simulink model "LMS_cs"  (R2023a)
settings: Solver=ode5  StartTime=0.0  StopTime=inf  FixedStep=1/200  RelTol=1e-3
PreLoadFcn:
  | mbxruntime.callbacks.PreLoadFcn(bdroot);
PostLoadFcn:
  | mbxruntime.callbacks.PostLoadFcn(bdroot);
InitFcn:
  | mbxruntime.callbacks.InitFcn(bdroot);
StartFcn:
  | mbxruntime.callbacks.StartFcn(bdroot);
StopFcn:
  | mbxruntime.callbacks.StopFcn(bdroot);
model workspace (MAT data in the model file):
  mbox_table : object (value not decoded)
  model_closed = 0
  sim_status = 0
undefined symbols (not defined in the file or in its folder): DiscIntNeverNeededParam, WheelL0, WheelL1, WheelR0, WheelR1
libraries: simulink x462, simulink_extras x117, PreScanSimulinkLibrary x33, PreScanUsefulBlocks x6, instrumentseriallib x5, simulink_need_slupdate x1
(part 62 of 68)

== system LMS_cs/BMW_X5_SUV_7/Dynamics_Simple_3D/Chassis/Bicycle_model_[XYZ]/X_Motion/BrakeSystem ==
  vx_[ms-1] : Inport
  BrakePressure_[bar] : Inport  Port=2
  Gain : Gain  Gain=1/p.Rw
  Saturation : Saturate  UpperLimit=p.PBrakeMax  LowerLimit=0
  Saturation1 : Saturate  UpperLimit=5/15  LowerLimit=-5/15
  Sign : Signum
  "[ms-1] 2 [rads-1]" : Gain  Gain=1/p.Rw  SaturateOnIntegerOverflow=on  OutDataTypeStr=Inherit: Same as input  ParamDataTypeStr=Inherit: Same as input
  braking Q factor : Gain  Gain=p.Qfac  SaturateOnIntegerOverflow=on  OutDataTypeStr=Inherit: Same as input  ParamDataTypeStr=Inherit: Same as input
  signed load1 : Product  InputSameDT=on  SaturateOnIntegerOverflow=on  OutDataTypeStr=Inherit: Same as first input
  BrakeForce : Outport
  BrakeTorqueAbs : Outport  Port=2
  wires:
  Gain/1 -> signed load1/1
  signed load1/1 -> BrakeForce/1
  Sign/1 -> signed load1/2  "sign"
  "[ms-1] 2 [rads-1]"/1 -> Saturation1/1
  Saturation1/1 -> Sign/1
  vx_[ms-1]/1 -> "[ms-1] 2 [rads-1]"/1
  Saturation/1 -> braking Q factor/1
  BrakePressure_[bar]/1 -> Saturation/1
  braking Q factor/1 -> Gain/1, BrakeTorqueAbs/1

== system LMS_cs/BMW_X5_SUV_7/Dynamics_Simple_3D/Chassis/Bicycle_model_[XYZ]/X_Motion/Configurable Subsystem ==
  In1 : Inport
  In2 : Inport  Port=2
  In3 : Inport  Port=3
  Integrator : Integrator  ExternalReset=level  InitialConditionSource=external
  Out1 : Outport
  wires:
  In1/1 -> Integrator/1
  In2/1 -> Integrator/2
  In3/1 -> Integrator/3
  Integrator/1 -> Out1/1

== system LMS_cs/BMW_X5_SUV_7/Dynamics_Simple_3D/Chassis/Bicycle_model_[XYZ]/X_Motion/Configurable Subsystem1 ==
  In1 : Inport
  Torsional damping : TransferFcn  Denominator=[0.1 1]
  Out1 : Outport
  wires:
  In1/1 -> Torsional damping/1
  Torsional damping/1 -> Out1/1

== system LMS_cs/BMW_X5_SUV_7/Dynamics_Simple_3D/Chassis/Bicycle_model_[XYZ]/X_Motion/Max RPM and zero- velocity detection ==
  note: Zero velocity detection
  note: Set to zero after infinite small time-step
  ax : Inport
  Drive Torque : Inport  Port=2
  Slope Torque : Inport  Port=3
  Brake Torque : Inport  Port=4
  v0 : Inport  Port=5
  vx : Inport  Port=6
  Abs : Abs  SaturateOnIntegerOverflow=off
  Abs1 : Abs  SaturateOnIntegerOverflow=off
  Compare To Zero : simulink/Logic and Bit Operations/Compare To Zero  relop=<=  OutDataTypeStr=boolean  ZeroCross=off
  Compare To Zero1 : simulink/Logic and Bit Operations/Compare To Zero  relop=>=  OutDataTypeStr=boolean  ZeroCross=off
  Compare To Zero2 : simulink/Logic and Bit Operations/Compare To Zero  relop=>=  OutDataTypeStr=boolean  ZeroCross=off
  Compare To Zero3 : simulink/Logic and Bit Operations/Compare To Zero  relop=<=  OutDataTypeStr=boolean  ZeroCross=off
  Configurable Subsystem : Subsystem  BlockChoice=Step  mask{ComputationMode=ComputationMode}
      mask prompts: ComputationMode "Compuation mode:"
      mask init:
      | SetComputationMode(gcb,ComputationMode);
      settings: AttributesFormatString=%<BlockChoice>  OpenFcn=BringToFront(gcb);  MemberBlocks=Discrete Step,Step
      settings: TemplateBlock=|
      | PreScanSimulinkLibrary/Configurable Subsystems/Step Function/Configurable
      | Subsystem
  Constant : Constant
  Constant1 : Constant
  Logical Operator : Logic  AllPortsSameDT=off  OutDataTypeStr=boolean
  Logical Operator1 : Logic  AllPortsSameDT=off  OutDataTypeStr=boolean
  Logical Operator2 : Logic  Operator=NOT  AllPortsSameDT=off  OutDataTypeStr=boolean
  Logical Operator3 : Logic  AllPortsSameDT=off  OutDataTypeStr=boolean
  Logical Operator4 : Logic  Operator=OR  AllPortsSameDT=off  OutDataTypeStr=boolean
  Memory : Memory
  Memory1 : Memory
  Memory2 : Memory
  Product : Product  RndMeth=Zero
  Relational Operator : RelationalOperator  Operator=<  OutDataTypeStr=boolean  InputSameDT=off
  SR-Memory : Subsystem
  Sum : Sum  Inputs=|-+
  Sum3 : Sum  InputSameDT=on  SaturateOnIntegerOverflow=on  OutDataTypeStr=Inherit: Same as first input
  Switch : Switch  Criteria=u2 ~= 0  Threshold=0.5  SaturateOnIntegerOverflow=off  InputSameDT=off
  ax is 0 : Constant  Value=0
  ax_out : Outport
  vx_reset : Outport  Port=2
  x0 : Outport  Port=3
  wires:
  Abs/1 -> Relational Operator/1
  Sum3/1 -> Abs/1
  Drive Torque/1 -> Sum3/1
  Slope Torque/1 -> Sum3/2
  Memory1/1 -> vx_reset/1  "vx"
  ax/1 -> Switch/1  "ax"
  Configurable Subsystem/1(Out1) -> Product/2
  Product/1 -> x0/1
  v0/1 -> Product/1
  Constant1/1 -> Sum/2
  ax is 0/1 -> Switch/3
  Sum/1 -> Switch/2
  Switch/1 -> ax_out/1
  SR-Memory/1(Out) -> Memory1/1, Sum/1
  Logical Operator2/1 -> SR-Memory/3(Reset)
  Constant/1 -> SR-Memory/1(Signal)
  Logical Operator1/1 -> SR-Memory/2(Set)
  Relational Operator/1 -> Logical Operator2/1, Logical Operator1/2
  Brake Torque/1 -> Abs1/1
  Abs1/1 -> Relational Operator/2
  Logical Operator/1 -> Logical Operator4/1  "zero-crossing forward"
  Compare To Zero1/1 -> Logical Operator/2
  Compare To Zero/1 -> Logical Operator/1
  Memory/1 -> Compare To Zero1/1
  Logical Operator3/1 -> Logical Operator4/2  "zero-crossing backward"
  Compare To Zero3/1 -> Logical Operator3/2
  Compare To Zero2/1 -> Logical Operator3/1
  Memory2/1 -> Compare To Zero3/1
  vx/1 -> Memory/1, Memory2/1, Compare To Zero2/1, Compare To Zero/1  "vx"
  Logical Operator4/1 -> Logical Operator1/1

== system LMS_cs/BMW_X5_SUV_7/Dynamics_Simple_3D/Chassis/Bicycle_model_[XYZ]/X_Motion/No contact rear wheels ==
  ForceIn [N] : Inport
  Compare To Zero : simulink/Logic and Bit Operations/Compare To Zero  relop=~=  OutDataTypeStr=boolean  ZeroCross=off
  Compare To Zero1 : simulink/Logic and Bit Operations/Compare To Zero  relop=~=  OutDataTypeStr=boolean  ZeroCross=off
  Constant : Constant  Value=0
  Logical Operator : Logic  AllPortsSameDT=off  OutDataTypeStr=boolean
  Switch : Switch  Criteria=u2 ~= 0  SaturateOnIntegerOverflow=off  InputSameDT=off
  ForceOut [N] : Outport
  wires:
  Switch/1 -> ForceOut [N]/1
  ForceIn [N]/1 -> Switch/1
  Logical Operator/1 -> Switch/2
  Compare To Zero1/1 -> Logical Operator/2
  Compare To Zero/1 -> Logical Operator/1
  [penetrationrearright] -> Compare To Zero1/1
  [penetrationrearleft] -> Compare To Zero/1
  Constant/1 -> Switch/3

== system LMS_cs/BMW_X5_SUV_7/Dynamics_Simple_3D/Chassis/Bicycle_model_[XYZ]/X_Motion/No contact wheels ==
  ForceIn [N] : Inport
  Brake repartition : Fcn  Expr=u(1) * (u(2)/4)
  Compare To Zero{,1..3} (4 alike) : simulink/Logic and Bit Operations/Compare To Zero  relop=~=  OutDataTypeStr=boolean  ZeroCross=off
  Mux : Mux  Inputs=[1 1 ]
  Sum : Sum  Inputs=++++  OutDataTypeStr=double
  ForceOut [N] : Outport
  wires:
  Brake repartition/1 -> ForceOut [N]/1
  Mux/1 -> Brake repartition/1
  Compare To Zero1/1 -> Sum/4
  Compare To Zero/1 -> Sum/3
  Compare To Zero3/1 -> Sum/2
  Compare To Zero2/1 -> Sum/1
  [penetrationfrontright] -> Compare To Zero3/1
  [penetrationfrontleft] -> Compare To Zero2/1
  ForceIn [N]/1 -> Mux/1
  Sum/1 -> Mux/2
  [penetrationrearright] -> Compare To Zero1/1
  [penetrationrearleft] -> Compare To Zero/1

== system LMS_cs/BMW_X5_SUV_7/Dynamics_Simple_3D/Chassis/Bicycle_model_[XYZ]/X_Motion/Slope Force ==
  slope_[rad] : Inport
  Fcn5 : Fcn  Expr=p.m*p.g*sin(u(1))
  SlopeForce_[N] : Outport
  wires:
  Fcn5/1 -> SlopeForce_[N]/1  "SlopeForce_[N]"
  slope_[rad]/1 -> Fcn5/1  "slope_[rad]"

== system LMS_cs/BMW_X5_SUV_7/Dynamics_Simple_3D/Chassis/Bicycle_model_[XYZ]/Y & Yaw_Motion/Configurable Subsystem ==
  In1 : Inport
  In2 : Inport  Port=2
  Integrator : Integrator  ExternalReset=level
  Out1 : Outport
  wires:
  In1/1 -> Integrator/1
  In2/1 -> Integrator/2
  Integrator/1 -> Out1/1

== system LMS_cs/BMW_X5_SUV_7/Dynamics_Simple_3D/Chassis/Bicycle_model_[XYZ]/Y & Yaw_Motion/Configurable Subsystem1 ==
  In1 : Inport
  In2 : Inport  Port=2
  Integrator : Integrator  ExternalReset=level
  Out1 : Outport
  wires:
  In1/1 -> Integrator/1
  In2/1 -> Integrator/2
  Integrator/1 -> Out1/1

== system LMS_cs/BMW_X5_SUV_7/Dynamics_Simple_3D/Chassis/Bicycle_model_[XYZ]/Y & Yaw_Motion/Configurable Subsystem2 ==
  In1 : Inport
  Integrator : Integrator
  Out1 : Outport
  wires:
  In1/1 -> Integrator/1
  Integrator/1 -> Out1/1

== system LMS_cs/BMW_X5_SUV_7/Dynamics_Simple_3D/Chassis/Bicycle_model_[XYZ]/Z, Pitch_Motion & Roll_Motion/Configurable Subsystem ==
  In1 : Inport
  Integrator : Integrator  LimitOutput=on  UpperSaturationLimit=25*pi/180  LowerSaturationLimit=-25*pi/180
  Out1 : Outport
  wires:
  In1/1 -> Integrator/1
  Integrator/1 -> Out1/1

== system LMS_cs/BMW_X5_SUV_7/Dynamics_Simple_3D/Chassis/Bicycle_model_[XYZ]/Z, Pitch_Motion & Roll_Motion/Configurable Subsystem1 ==
  In1 : Inport
  Integrator : Integrator
  Out1 : Outport
  wires:
  In1/1 -> Integrator/1
  Integrator/1 -> Out1/1

== system LMS_cs/BMW_X5_SUV_7/Dynamics_Simple_3D/Chassis/Bicycle_model_[XYZ]/Z, Pitch_Motion & Roll_Motion/Configurable Subsystem2 ==
  In1 : Inport
  Integrator : Integrator
  Out1 : Outport
  wires:
  In1/1 -> Integrator/1
  Integrator/1 -> Out1/1

== system LMS_cs/BMW_X5_SUV_7/Dynamics_Simple_3D/Chassis/Bicycle_model_[XYZ]/Z, Pitch_Motion & Roll_Motion/Configurable Subsystem3 ==
  In1 : Inport
  Integrator : Integrator
  Out1 : Outport
  wires:
  In1/1 -> Integrator/1
  Integrator/1 -> Out1/1

== system LMS_cs/BMW_X5_SUV_7/Dynamics_Simple_3D/Chassis/Bicycle_model_[XYZ]/Z, Pitch_Motion & Roll_Motion/Configurable Subsystem4 ==
  In1 : Inport
  Integrator : Integrator
  Out1 : Outport
  wires:
  In1/1 -> Integrator/1
  Integrator/1 -> Out1/1

== system LMS_cs/BMW_X5_SUV_7/Dynamics_Simple_3D/Chassis/Bicycle_model_[XYZ]/Z, Pitch_Motion & Roll_Motion/Configurable Subsystem5 ==
  In1 : Inport
  Derivative : Derivative
  Out1 : Outport
  wires:
  In1/1 -> Derivative/1
  Derivative/1 -> Out1/1

== system LMS_cs/BMW_X5_SUV_7/Dynamics_Simple_3D/Chassis/Bicycle_model_[XYZ]/Z, Pitch_Motion & Roll_Motion/Configurable Subsystem6 ==
  In1 : Inport
  Derivative : Derivative
  Out1 : Outport
  wires:
  In1/1 -> Derivative/1
  Derivative/1 -> Out1/1

== system LMS_cs/BMW_X5_SUV_7/Dynamics_Simple_3D/Chassis/Bicycle_model_[XYZ]/Z, Pitch_Motion & Roll_Motion/Configurable Subsystem7 ==
  In1 : Inport
  Derivative : Derivative
  Out1 : Outport
  wires:
  In1/1 -> Derivative/1
  Derivative/1 -> Out1/1

== system LMS_cs/BMW_X5_SUV_7/Dynamics_Simple_3D/Chassis/Bicycle_model_[XYZ]/Z, Pitch_Motion & Roll_Motion/Configurable Subsystem8 ==
  In1 : Inport
  Derivative : Derivative
  Out1 : Outport
  wires:
  In1/1 -> Derivative/1
  Derivative/1 -> Out1/1

== system LMS_cs/BMW_X5_SUV_7/Dynamics_Simple_3D/Chassis/Bicycle_model_[XYZ]/Z, Pitch_Motion & Roll_Motion/Configurable Subsystem9 ==
  In1 : Inport
  Derivative : Derivative
  Out1 : Outport
  wires:
  In1/1 -> Derivative/1
  Derivative/1 -> Out1/1

== system LMS_cs/BMW_X5_SUV_7/Dynamics_Simple_3D/Chassis/Bicycle_model_[XYZ]/Z_Motion unsprung mass/Configurable Subsystem ==
  In1 : Inport
  Derivative : Derivative
  Out1 : Outport
  wires:
  In1/1 -> Derivative/1
  Derivative/1 -> Out1/1

== system LMS_cs/BMW_X5_SUV_7/Dynamics_Simple_3D/Chassis/Bicycle_model_[XYZ]/Z_Motion unsprung mass/Configurable Subsystem1 ==
  In1 : Inport
  Integrator : Integrator
  Out1 : Outport
  wires:
  In1/1 -> Integrator/1
  Integrator/1 -> Out1/1

== system LMS_cs/BMW_X5_SUV_7/Dynamics_Simple_3D/Chassis/Bicycle_model_[XYZ]/Z_Motion unsprung mass/Configurable Subsystem10 ==
  In1 : Inport
  Derivative : Derivative
  Out1 : Outport
  wires:
  In1/1 -> Derivative/1
  Derivative/1 -> Out1/1

== system LMS_cs/BMW_X5_SUV_7/Dynamics_Simple_3D/Chassis/Bicycle_model_[XYZ]/Z_Motion unsprung mass/Configurable Subsystem11 ==
  In1 : Inport
  Derivative : Derivative
  Out1 : Outport
  wires:
  In1/1 -> Derivative/1
  Derivative/1 -> Out1/1

== system LMS_cs/BMW_X5_SUV_7/Dynamics_Simple_3D/Chassis/Bicycle_model_[XYZ]/Z_Motion unsprung mass/Configurable Subsystem2 ==
  In1 : Inport
  Integrator : Integrator
  Out1 : Outport
  wires:
  In1/1 -> Integrator/1
  Integrator/1 -> Out1/1

== system LMS_cs/BMW_X5_SUV_7/Dynamics_Simple_3D/Chassis/Bicycle_model_[XYZ]/Z_Motion unsprung mass/Configurable Subsystem3 ==
  In1 : Inport
  Integrator : Integrator
  Out1 : Outport
  wires:
  In1/1 -> Integrator/1
  Integrator/1 -> Out1/1

== system LMS_cs/BMW_X5_SUV_7/Dynamics_Simple_3D/Chassis/Bicycle_model_[XYZ]/Z_Motion unsprung mass/Configurable Subsystem4 ==
  In1 : Inport
  Integrator : Integrator
  Out1 : Outport
  wires:
  In1/1 -> Integrator/1
  Integrator/1 -> Out1/1

== system LMS_cs/BMW_X5_SUV_7/Dynamics_Simple_3D/Chassis/Bicycle_model_[XYZ]/Z_Motion unsprung mass/Configurable Subsystem5 ==
  In1 : Inport
  Integrator : Integrator
  Out1 : Outport
  wires:
  In1/1 -> Integrator/1
  Integrator/1 -> Out1/1

== system LMS_cs/BMW_X5_SUV_7/Dynamics_Simple_3D/Chassis/Bicycle_model_[XYZ]/Z_Motion unsprung mass/Configurable Subsystem6 ==
  In1 : Inport
  Integrator : Integrator
  Out1 : Outport
  wires:
  In1/1 -> Integrator/1
  Integrator/1 -> Out1/1

== system LMS_cs/BMW_X5_SUV_7/Dynamics_Simple_3D/Chassis/Bicycle_model_[XYZ]/Z_Motion unsprung mass/Configurable Subsystem7 ==
  In1 : Inport
  Integrator : Integrator
  Out1 : Outport
  wires:
  In1/1 -> Integrator/1
  Integrator/1 -> Out1/1

== system LMS_cs/BMW_X5_SUV_7/Dynamics_Simple_3D/Chassis/Bicycle_model_[XYZ]/Z_Motion unsprung mass/Configurable Subsystem8 ==
  In1 : Inport
  Integrator : Integrator
  Out1 : Outport
  wires:
  In1/1 -> Integrator/1
  Integrator/1 -> Out1/1

== system LMS_cs/BMW_X5_SUV_7/Dynamics_Simple_3D/Chassis/Bicycle_model_[XYZ]/Z_Motion unsprung mass/Configurable Subsystem9 ==
  In1 : Inport
  Derivative : Derivative
  Out1 : Outport
  wires:
  In1/1 -> Derivative/1
  Derivative/1 -> Out1/1

== system LMS_cs/BMW_X5_SUV_7/Dynamics_Simple_3D/Chassis/FrontTyre/AlphaFront/Enabled Subsystem ==
  In : Inport
  Enable : EnablePort  PropagateVarSize=During execution
  AlphaFront : Fcn  Expr=-atan( (u(2)+u(3)*p.a)/u(1) )
  Alpha : Outport  OutputWhenDisabled=reset  InitialOutput=[0]
  wires:
  AlphaFront/1 -> Alpha/1
  In/1 -> AlphaFront/1

== system LMS_cs/BMW_X5_SUV_7/Dynamics_Simple_3D/Chassis/RearTyre/AlphaRear/Enabled Subsystem ==
  In : Inport
  Enable : EnablePort  PropagateVarSize=During execution
  AlphaRear : Fcn  Expr=-atan( (u(2)-u(3)*p.b)/u(1) )
  Alpha : Outport  OutputWhenDisabled=reset  InitialOutput=[0]
  wires:
  AlphaRear/1 -> Alpha/1
  In/1 -> AlphaRear/1

== system LMS_cs/BMW_X5_SUV_7/PreScan_Contact_Sensor/Vehicle Local to World/state2FullState/limit roll/Substitute 90 & 270 deg (and its plurals) ==
  Angle [rad] : Inport
  270 deg detection : simulink/Model Verification/Check  Static Gap  Description=u <= 269.5 || 270.5 <= u  max=270.5  max_included=on  min=269.5  min_included=on  enabled=on  stopWhenAssertionFail=off  export=on  icon=graphic
  90 deg detection : simulink/Model Verification/Check  Static Gap  Description=u <= 89.5 || 90.5 <= u  max=90.5  max_included=on  min=89.5  min_included=on  enabled=on  stopWhenAssertionFail=off  export=on  icon=graphic
  Angle 0-360 deg limiter : Subsystem
  Degrees to Radians : simulink_extras/Transformations/Degrees to Radians
  Radians to Degrees : simulink_extras/Transformations/Radians to Degrees
  Substitution Value : Constant  Value=269.5
  Substitution Value : Constant  Value=89.5
  Switch : Switch  Threshold=0.5  SaturateOnIntegerOverflow=off  InputSameDT=off
  Switch1 : Switch  Threshold=0.5  SaturateOnIntegerOverflow=off  InputSameDT=off
  Subst Angle [rad] : Outport
  wires:
  Angle [rad]/1 -> Radians to Degrees/1
  Degrees to Radians/1 -> Subst Angle [rad]/1
  Radians to Degrees/1 -> Angle 0-360 deg limiter/1(Angle [deg])
  Switch1/1 -> Degrees to Radians/1
  Substitution Value/1 -> Switch1/3
  270 deg detection/1 -> Switch1/2
  Switch/1 -> Switch1/1, 270 deg detection/1
  Substitution Value/1 -> Switch/3
  90 deg detection/1 -> Switch/2
  Angle 0-360 deg limiter/1(LimAngle [deg]) -> 90 deg detection/1, Switch/1

== system LMS_cs/BMW_X5_SUV_8/Dynamics_Simple_3D/Chassis/Bicycle_model_[XYZ]/RoadContact/Penetration depth ==
  TyreInfo_in : Inport
  Bus Selector1 : BusSelector  OutputSignals=TireFL.cp0.penetrationdepth,TireFL.cp0.normal.z,TireFL.cp1.penetrationdepth,TireFL.cp1.normal.z,TireFL.cp2.penetrationdepth,TireFL.cp2.normal.z,TireFL.cp3.penetrationdepth,TireFL.cp3.normal.z,TireFR.cp0.penetrationdepth,TireFR.cp0.normal.z,TireFR.cp1.penetrationdepth,TireFR.cp1.normal.z,TireFR.cp2.penetrationdepth,TireFR.cp2.normal.z,TireFR.cp3.penetrationdepth,TireFR.cp3.normal.z,TireRL.cp0.penetrationdepth,TireRL.cp0.normal.z,TireRL.cp1.penetrationdepth,TireRL.cp1.normal.z,TireRL.cp2.penetrationdepth,TireRL.cp2.normal.z,TireRL.cp3.penetrationdepth,TireRL.cp3.normal.z,TireRR.cp0.penetrationdepth,TireRR.cp0.normal.z,TireRR.cp1.penetrationdepth,TireRR.cp1.normal.z,TireRR.cp2.penetrationdepth,TireRR.cp2.normal.z,TireRR.cp3.penetrationdepth,TireRR.cp3.normal.z
  Fcn{,1..15} (16 alike) : Fcn  Expr=u(1)*u(2)
  MinMax{1..4} (4 alike) : MinMax
  Mux{1..4} (4 alike) : Mux
  Mux{5..20} (16 alike) : Mux  Inputs=2
  Saturation{1..4} (4 alike) : Saturate  UpperLimit=0  LowerLimit=-inf
  depth_FL [m] : Outport
  depth_FR [m] : Outport  Port=2
  depth_RL [m] : Outport  Port=3
  depth_RR [m] : Outport  Port=4
  wires:
  Fcn15/1 -> Mux4/4
  Fcn14/1 -> Mux4/3
  Fcn13/1 -> Mux4/2
  Fcn12/1 -> Mux4/1
  Fcn11/1 -> Mux2/4
  Fcn10/1 -> Mux2/3
  Fcn9/1 -> Mux2/2
  Fcn8/1 -> Mux2/1
  Mux15/1 -> Fcn15/1
  Mux14/1 -> Fcn14/1
  Mux13/1 -> Fcn13/1
  Mux20/1 -> Fcn12/1
  Mux19/1 -> Fcn11/1
  Mux18/1 -> Fcn10/1
  Mux17/1 -> Fcn9/1
  Mux16/1 -> Fcn8/1
  Fcn7/1 -> Mux1/4
  Fcn6/1 -> Mux1/3
  Fcn5/1 -> Mux1/2
  Fcn4/1 -> Mux1/1
  Fcn3/1 -> Mux3/4
  Fcn2/1 -> Mux3/3
  Fcn1/1 -> Mux3/2
  Fcn/1 -> Mux3/1
  Mux12/1 -> Fcn7/1
  Mux11/1 -> Fcn6/1
  Mux10/1 -> Fcn5/1
  Mux9/1 -> Fcn4/1
  Mux8/1 -> Fcn3/1
  Mux7/1 -> Fcn2/1
  Mux6/1 -> Fcn1/1
  Mux5/1 -> Fcn/1
  MinMax1/1 -> Saturation2/1
  Mux1/1 -> MinMax1/1
  MinMax2/1 -> Saturation3/1
  Mux2/1 -> MinMax2/1
  MinMax4/1 -> Saturation1/1
  Bus Selector1/32 -> Mux15/2  "<z>"
  Bus Selector1/31 -> Mux15/1  "<penetrationdepth>"
  Bus Selector1/30 -> Mux14/2  "<z>"
  Bus Selector1/29 -> Mux14/1  "<penetrationdepth>"
  Bus Selector1/28 -> Mux13/2  "<z>"
  Bus Selector1/27 -> Mux13/1  "<penetrationdepth>"
  Bus Selector1/26 -> Mux20/2  "<z>"
  Bus Selector1/25 -> Mux20/1  "<penetrationdepth>"
  Bus Selector1/24 -> Mux19/2  "<z>"
  Bus Selector1/23 -> Mux19/1  "<penetrationdepth>"
  Bus Selector1/22 -> Mux18/2  "<z>"
  Bus Selector1/21 -> Mux18/1  "<penetrationdepth>"
  Bus Selector1/20 -> Mux17/2  "<z>"
  Bus Selector1/19 -> Mux17/1  "<penetrationdepth>"
  Bus Selector1/18 -> Mux16/2  "<z>"
  Bus Selector1/17 -> Mux16/1  "<penetrationdepth>"
  Bus Selector1/16 -> Mux12/2  "<z>"
  Bus Selector1/15 -> Mux12/1  "<penetrationdepth>"
  Bus Selector1/14 -> Mux11/2  "<z>"
  Bus Selector1/13 -> Mux11/1  "<penetrationdepth>"
  Bus Selector1/12 -> Mux10/2  "<z>"
  Bus Selector1/11 -> Mux10/1  "<penetrationdepth>"
  Bus Selector1/10 -> Mux9/2  "<z>"
  Bus Selector1/9 -> Mux9/1  "<penetrationdepth>"
  Bus Selector1/8 -> Mux8/2  "<z>"
  Bus Selector1/7 -> Mux8/1  "<penetrationdepth>"
  Bus Selector1/6 -> Mux7/2  "<z>"
  Bus Selector1/5 -> Mux7/1  "<penetrationdepth>"
  Bus Selector1/4 -> Mux6/2  "<z>"
  Bus Selector1/3 -> Mux6/1  "<penetrationdepth>"
  Bus Selector1/2 -> Mux5/2  "<z>"
  Bus Selector1/1 -> Mux5/1  "<penetrationdepth>"
  Mux4/1 -> MinMax3/1
  MinMax3/1 -> Saturation4/1
  Mux3/1 -> MinMax4/1
  Saturation1/1 -> depth_FL [m]/1
  Saturation2/1 -> depth_FR [m]/1
  TyreInfo_in/1 -> Bus Selector1/1
  Saturation3/1 -> depth_RL [m]/1
  Saturation4/1 -> depth_RR [m]/1

== system LMS_cs/BMW_X5_SUV_8/Dynamics_Simple_3D/Chassis/Bicycle_model_[XYZ]/RoadContact/RoadGeometry ==
  TyreInfo_in : Inport
  Calc_banking : Subsystem
  Calc_slope : Subsystem
  Calc_z : Subsystem
  DocBlock : simulink/Model-Wide Utilities/DocBlock  DocumentType=Text
      content=|
      | This block determines, based on the z-coordinates of the road in
      | correspondence of the contact points,
      | - the z-coordinate of the road in correspondence of the middle point of the
      |   vehicle (z);
      | - the slope angle of the road (alpha, positive when downhill);
      | - the banking angle of the road (beta, positive when counter-clockwise when
      |   looking from the front of the vehicle).
      |
      | For every wheel there are 4 contact points (cp0, cp1, cp2, cp3) defined in
      | TyreInfo_in. Not all 4 contact points reports always a value, depending on
      | different conditions there might be contact points that do not report a
      | value. These points report in this case to 0. If the tyre is lifted from
      | the road, all contact points report 0. Because of this reason, the
      | value of the contact point that reports the largest negative value of the
      | penetration depth is used. If all values of the penetration depth are 0,
      | then a maximum gradient is applied to avoid jumps to 0 in the z signal.
      | The maximum gradient is fixed to -6 [m/s^2], this value is large enough for
      | a vehicle driving at 30 [m/s] downhill on a gradient of 20 [%]. Further, a
      | first order low pass linear filter with a bandwidth of 1 [Hz] is applied.
      | This filter removes high frequencies components in the signal, when one
      | wheel is lifted (e.g. drive in a corner with a large lateral acceleration).
      | The bandwidth of 1 [Hz] is large enough to include the main frequencies
      | that occurr in the vehicle roll, pitch and vertical movements.
      |
      | z, slope and banking are determined as follows:
      |
      | z        = (+ zFL + zFR + zRL + zRR) / 4            (Calc_z)
      | slope    = (- zFL - zFR + zRL + zRR) / (2*p.l)      (Calc_slope)
      | banking  = (+ zFL - zFR + zRL - zRR) / (2*p.width)  (Calc_banking)
  Mux4 : Mux
  zFL_lowerpenetrationdetph : Subsystem
  zFL_tyreinfo : Subsystem
  zFR_lowerpenetrationdetph : Subsystem
  zFR_tyreinfo : Subsystem
  zRL_lowerpenetrationdetph : Subsystem
  zRL_tyreinfo : Subsystem
  zRR_lowerpenetrationdetph : Subsystem
  zRR_tyreinfo : Subsystem
  z : Outport
  slope : Outport  Port=2
  banking : Outport  Port=3
  wires:
  TyreInfo_in/1 -> zFL_tyreinfo/1(In1), zFR_tyreinfo/1(In1), zRL_tyreinfo/1(In1), zRR_tyreinfo/1(In1)
  Calc_z/1(z) -> z/1
  Mux4/1 -> Calc_z/1(zi), Calc_slope/1(zi), Calc_banking/1(zi)
  Calc_slope/1(slope) -> slope/1
  Calc_banking/1(banking) -> banking/1
  zFL_lowerpenetrationdetph/1(z) -> Mux4/1
  zFR_lowerpenetrationdetph/1(z) -> Mux4/2
  zRL_lowerpenetrationdetph/1(z) -> Mux4/3
  zRR_lowerpenetrationdetph/1(z) -> Mux4/4
  zFL_tyreinfo/1(penetrationdepth) -> zFL_lowerpenetrationdetph/1(penetrationdepth)
  zFL_tyreinfo/2(position_z) -> zFL_lowerpenetrationdetph/2(position_z)
  zFL_tyreinfo/3(normal_z) -> zFL_lowerpenetrationdetph/3(normal_z)
  zFR_tyreinfo/1(penetrationdepth) -> zFR_lowerpenetrationdetph/1(penetrationdepth)
  zFR_tyreinfo/2(position_z) -> zFR_lowerpenetrationdetph/2(position_z)
  zFR_tyreinfo/3(normal_z) -> zFR_lowerpenetrationdetph/3(normal_z)
  zRL_tyreinfo/1(penetrationdepth) -> zRL_lowerpenetrationdetph/1(penetrationdepth)
  zRL_tyreinfo/2(position_z) -> zRL_lowerpenetrationdetph/2(position_z)
  zRL_tyreinfo/3(normal_z) -> zRL_lowerpenetrationdetph/3(normal_z)
  zRR_tyreinfo/1(penetrationdepth) -> zRR_lowerpenetrationdetph/1(penetrationdepth)
  zRR_tyreinfo/2(position_z) -> zRR_lowerpenetrationdetph/2(position_z)
  zRR_tyreinfo/3(normal_z) -> zRR_lowerpenetrationdetph/3(normal_z)

== system LMS_cs/BMW_X5_SUV_8/Dynamics_Simple_3D/Chassis/Bicycle_model_[XYZ]/X_Motion/Air&RoadResistance ==
  vx_[ms-1] : Inport
  slope_[rad] : Inport  Port=2
  Gain : Gain  Gain=1/p.Rw
  Mux4 : Mux  Inputs=2
  Road & Aerodyn Resistances : Fcn  Expr=p.Rroad*cos(u(2)) + p.Rair*u(1)^2
  Saturation1 : Saturate  UpperLimit=5/15  LowerLimit=-5/15
  Sign : Signum
  "[ms-1] 2 [rads-1]" : Gain  Gain=1/p.Rw  SaturateOnIntegerOverflow=on  OutDataTypeStr=Inherit: Same as input  ParamDataTypeStr=Inherit: Same as input
  signed load1 : Product  InputSameDT=on  SaturateOnIntegerOverflow=on  OutDataTypeStr=Inherit: Same as first input
  Resistance_Force : Outport
  wires:
  Gain/1 -> signed load1/1  "ResistanceForce_[N]"
  slope_[rad]/1 -> Mux4/2
  Mux4/1 -> Road & Aerodyn Resistances/1
  Road & Aerodyn Resistances/1 -> Gain/1  "ResistanceTorque_[Nm]"
  Sign/1 -> signed load1/2  "sign"
  "[ms-1] 2 [rads-1]"/1 -> Saturation1/1
  Saturation1/1 -> Sign/1
  vx_[ms-1]/1 -> Mux4/1, "[ms-1] 2 [rads-1]"/1
  signed load1/1 -> Resistance_Force/1  "F_[N]"

== system LMS_cs/BMW_X5_SUV_8/Dynamics_Simple_3D/Chassis/Bicycle_model_[XYZ]/X_Motion/BrakeSystem ==
  vx_[ms-1] : Inport
  BrakePressure_[bar] : Inport  Port=2
  Gain : Gain  Gain=1/p.Rw
  Saturation : Saturate  UpperLimit=p.PBrakeMax  LowerLimit=0
  Saturation1 : Saturate  UpperLimit=5/15  LowerLimit=-5/15
  Sign : Signum
  "[ms-1] 2 [rads-1]" : Gain  Gain=1/p.Rw  SaturateOnIntegerOverflow=on  OutDataTypeStr=Inherit: Same as input  ParamDataTypeStr=Inherit: Same as input
  braking Q factor : Gain  Gain=p.Qfac  SaturateOnIntegerOverflow=on  OutDataTypeStr=Inherit: Same as input  ParamDataTypeStr=Inherit: Same as input
  signed load1 : Product  InputSameDT=on  SaturateOnIntegerOverflow=on  OutDataTypeStr=Inherit: Same as first input
  BrakeForce : Outport
  BrakeTorqueAbs : Outport  Port=2
  wires:
  Gain/1 -> signed load1/1
  signed load1/1 -> BrakeForce/1
  Sign/1 -> signed load1/2  "sign"
  "[ms-1] 2 [rads-1]"/1 -> Saturation1/1
  Saturation1/1 -> Sign/1
  vx_[ms-1]/1 -> "[ms-1] 2 [rads-1]"/1
  Saturation/1 -> braking Q factor/1
  BrakePressure_[bar]/1 -> Saturation/1
  braking Q factor/1 -> Gain/1, BrakeTorqueAbs/1

== system LMS_cs/BMW_X5_SUV_8/Dynamics_Simple_3D/Chassis/Bicycle_model_[XYZ]/X_Motion/Configurable Subsystem ==
  In1 : Inport
  In2 : Inport  Port=2
  In3 : Inport  Port=3
  Integrator : Integrator  ExternalReset=level  InitialConditionSource=external
  Out1 : Outport
  wires:
  In1/1 -> Integrator/1
  In2/1 -> Integrator/2
  In3/1 -> Integrator/3
  Integrator/1 -> Out1/1

== system LMS_cs/BMW_X5_SUV_8/Dynamics_Simple_3D/Chassis/Bicycle_model_[XYZ]/X_Motion/Configurable Subsystem1 ==
  In1 : Inport
  Torsional damping : TransferFcn  Denominator=[0.1 1]
  Out1 : Outport
  wires:
  In1/1 -> Torsional damping/1
  Torsional damping/1 -> Out1/1

== system LMS_cs/BMW_X5_SUV_8/Dynamics_Simple_3D/Chassis/Bicycle_model_[XYZ]/X_Motion/Max RPM and zero- velocity detection ==
  note: Zero velocity detection
  note: Set to zero after infinite small time-step
  ax : Inport
  Drive Torque : Inport  Port=2
  Slope Torque : Inport  Port=3
  Brake Torque : Inport  Port=4
  v0 : Inport  Port=5
  vx : Inport  Port=6
  Abs : Abs  SaturateOnIntegerOverflow=off
  Abs1 : Abs  SaturateOnIntegerOverflow=off
  Compare To Zero : simulink/Logic and Bit Operations/Compare To Zero  relop=<=  OutDataTypeStr=boolean  ZeroCross=off
  Compare To Zero1 : simulink/Logic and Bit Operations/Compare To Zero  relop=>=  OutDataTypeStr=boolean  ZeroCross=off
  Compare To Zero2 : simulink/Logic and Bit Operations/Compare To Zero  relop=>=  OutDataTypeStr=boolean  ZeroCross=off
  Compare To Zero3 : simulink/Logic and Bit Operations/Compare To Zero  relop=<=  OutDataTypeStr=boolean  ZeroCross=off
  Configurable Subsystem : Subsystem  BlockChoice=Step  mask{ComputationMode=ComputationMode}
      mask prompts: ComputationMode "Compuation mode:"
      mask init:
      | SetComputationMode(gcb,ComputationMode);
      settings: AttributesFormatString=%<BlockChoice>  OpenFcn=BringToFront(gcb);  MemberBlocks=Discrete Step,Step
      settings: TemplateBlock=|
      | PreScanSimulinkLibrary/Configurable Subsystems/Step Function/Configurable
      | Subsystem
  Constant : Constant
  Constant1 : Constant
  Logical Operator : Logic  AllPortsSameDT=off  OutDataTypeStr=boolean
  Logical Operator1 : Logic  AllPortsSameDT=off  OutDataTypeStr=boolean
  Logical Operator2 : Logic  Operator=NOT  AllPortsSameDT=off  OutDataTypeStr=boolean
  Logical Operator3 : Logic  AllPortsSameDT=off  OutDataTypeStr=boolean
  Logical Operator4 : Logic  Operator=OR  AllPortsSameDT=off  OutDataTypeStr=boolean
  Memory : Memory
  Memory1 : Memory
  Memory2 : Memory
  Product : Product  RndMeth=Zero
  Relational Operator : RelationalOperator  Operator=<  OutDataTypeStr=boolean  InputSameDT=off
  SR-Memory : Subsystem
  Sum : Sum  Inputs=|-+
  Sum3 : Sum  InputSameDT=on  SaturateOnIntegerOverflow=on  OutDataTypeStr=Inherit: Same as first input
  Switch : Switch  Criteria=u2 ~= 0  Threshold=0.5  SaturateOnIntegerOverflow=off  InputSameDT=off
  ax is 0 : Constant  Value=0
  ax_out : Outport
  vx_reset : Outport  Port=2
  x0 : Outport  Port=3
  wires:
  Abs/1 -> Relational Operator/1
  Sum3/1 -> Abs/1
  Drive Torque/1 -> Sum3/1
  Slope Torque/1 -> Sum3/2
  Memory1/1 -> vx_reset/1  "vx"
  ax/1 -> Switch/1  "ax"
  Configurable Subsystem/1(Out1) -> Product/2
  Product/1 -> x0/1
  v0/1 -> Product/1
  Constant1/1 -> Sum/2
  ax is 0/1 -> Switch/3
  Sum/1 -> Switch/2
  Switch/1 -> ax_out/1
  SR-Memory/1(Out) -> Memory1/1, Sum/1
  Logical Operator2/1 -> SR-Memory/3(Reset)
  Constant/1 -> SR-Memory/1(Signal)
  Logical Operator1/1 -> SR-Memory/2(Set)
  Relational Operator/1 -> Logical Operator2/1, Logical Operator1/2
  Brake Torque/1 -> Abs1/1
  Abs1/1 -> Relational Operator/2
  Logical Operator/1 -> Logical Operator4/1  "zero-crossing forward"
  Compare To Zero1/1 -> Logical Operator/2
  Compare To Zero/1 -> Logical Operator/1
  Memory/1 -> Compare To Zero1/1
  Logical Operator3/1 -> Logical Operator4/2  "zero-crossing backward"
  Compare To Zero3/1 -> Logical Operator3/2
  Compare To Zero2/1 -> Logical Operator3/1
  Memory2/1 -> Compare To Zero3/1
  vx/1 -> Memory/1, Memory2/1, Compare To Zero2/1, Compare To Zero/1  "vx"
  Logical Operator4/1 -> Logical Operator1/1

== system LMS_cs/BMW_X5_SUV_8/Dynamics_Simple_3D/Chassis/Bicycle_model_[XYZ]/X_Motion/No contact rear wheels ==
  ForceIn [N] : Inport
  Compare To Zero : simulink/Logic and Bit Operations/Compare To Zero  relop=~=  OutDataTypeStr=boolean  ZeroCross=off
  Compare To Zero1 : simulink/Logic and Bit Operations/Compare To Zero  relop=~=  OutDataTypeStr=boolean  ZeroCross=off
  Constant : Constant  Value=0
  Logical Operator : Logic  AllPortsSameDT=off  OutDataTypeStr=boolean
  Switch : Switch  Criteria=u2 ~= 0  SaturateOnIntegerOverflow=off  InputSameDT=off
  ForceOut [N] : Outport
  wires:
  Switch/1 -> ForceOut [N]/1
  ForceIn [N]/1 -> Switch/1
  Logical Operator/1 -> Switch/2
  Compare To Zero1/1 -> Logical Operator/2
  Compare To Zero/1 -> Logical Operator/1
  [penetrationrearright] -> Compare To Zero1/1
  [penetrationrearleft] -> Compare To Zero/1
  Constant/1 -> Switch/3

== system LMS_cs/BMW_X5_SUV_8/Dynamics_Simple_3D/Chassis/Bicycle_model_[XYZ]/X_Motion/No contact wheels ==
  ForceIn [N] : Inport
  Brake repartition : Fcn  Expr=u(1) * (u(2)/4)
  Compare To Zero{,1..3} (4 alike) : simulink/Logic and Bit Operations/Compare To Zero  relop=~=  OutDataTypeStr=boolean  ZeroCross=off
  Mux : Mux  Inputs=[1 1 ]
  Sum : Sum  Inputs=++++  OutDataTypeStr=double
  ForceOut [N] : Outport
  wires:
  Brake repartition/1 -> ForceOut [N]/1
  Mux/1 -> Brake repartition/1
  Compare To Zero1/1 -> Sum/4
  Compare To Zero/1 -> Sum/3
  Compare To Zero3/1 -> Sum/2
  Compare To Zero2/1 -> Sum/1
  [penetrationfrontright] -> Compare To Zero3/1
  [penetrationfrontleft] -> Compare To Zero2/1
  ForceIn [N]/1 -> Mux/1
  Sum/1 -> Mux/2
  [penetrationrearright] -> Compare To Zero1/1
  [penetrationrearleft] -> Compare To Zero/1

== system LMS_cs/BMW_X5_SUV_8/Dynamics_Simple_3D/Chassis/Bicycle_model_[XYZ]/X_Motion/Slope Force ==
  slope_[rad] : Inport
  Fcn5 : Fcn  Expr=p.m*p.g*sin(u(1))
  SlopeForce_[N] : Outport
  wires:
  Fcn5/1 -> SlopeForce_[N]/1  "SlopeForce_[N]"
  slope_[rad]/1 -> Fcn5/1  "slope_[rad]"

== system LMS_cs/BMW_X5_SUV_8/Dynamics_Simple_3D/Chassis/Bicycle_model_[XYZ]/Y & Yaw_Motion/Configurable Subsystem ==
  In1 : Inport
  In2 : Inport  Port=2
  Integrator : Integrator  ExternalReset=level
  Out1 : Outport
  wires:
  In1/1 -> Integrator/1
  In2/1 -> Integrator/2
  Integrator/1 -> Out1/1

== system LMS_cs/BMW_X5_SUV_8/Dynamics_Simple_3D/Chassis/Bicycle_model_[XYZ]/Y & Yaw_Motion/Configurable Subsystem1 ==
  In1 : Inport
  In2 : Inport  Port=2
  Integrator : Integrator  ExternalReset=level
  Out1 : Outport
  wires:
  In1/1 -> Integrator/1
  In2/1 -> Integrator/2
  Integrator/1 -> Out1/1

== system LMS_cs/BMW_X5_SUV_8/Dynamics_Simple_3D/Chassis/Bicycle_model_[XYZ]/Y & Yaw_Motion/Configurable Subsystem2 ==
  In1 : Inport
  Integrator : Integrator
  Out1 : Outport
  wires:
  In1/1 -> Integrator/1
  Integrator/1 -> Out1/1

== system LMS_cs/BMW_X5_SUV_8/Dynamics_Simple_3D/Chassis/Bicycle_model_[XYZ]/Z, Pitch_Motion & Roll_Motion/Configurable Subsystem ==
  In1 : Inport
  Integrator : Integrator  LimitOutput=on  UpperSaturationLimit=25*pi/180  LowerSaturationLimit=-25*pi/180
  Out1 : Outport
  wires:
  In1/1 -> Integrator/1
  Integrator/1 -> Out1/1

== system LMS_cs/BMW_X5_SUV_8/Dynamics_Simple_3D/Chassis/Bicycle_model_[XYZ]/Z, Pitch_Motion & Roll_Motion/Configurable Subsystem1 ==
  In1 : Inport
  Integrator : Integrator
  Out1 : Outport
  wires:
  In1/1 -> Integrator/1
  Integrator/1 -> Out1/1

== system LMS_cs/BMW_X5_SUV_8/Dynamics_Simple_3D/Chassis/Bicycle_model_[XYZ]/Z, Pitch_Motion & Roll_Motion/Configurable Subsystem2 ==
  In1 : Inport
  Integrator : Integrator
  Out1 : Outport
  wires:
  In1/1 -> Integrator/1
  Integrator/1 -> Out1/1

== system LMS_cs/BMW_X5_SUV_8/Dynamics_Simple_3D/Chassis/Bicycle_model_[XYZ]/Z, Pitch_Motion & Roll_Motion/Configurable Subsystem3 ==
  In1 : Inport
  Integrator : Integrator
  Out1 : Outport
  wires:
  In1/1 -> Integrator/1
  Integrator/1 -> Out1/1

== system LMS_cs/BMW_X5_SUV_8/Dynamics_Simple_3D/Chassis/Bicycle_model_[XYZ]/Z, Pitch_Motion & Roll_Motion/Configurable Subsystem4 ==
  In1 : Inport
  Integrator : Integrator
  Out1 : Outport
  wires:
  In1/1 -> Integrator/1
  Integrator/1 -> Out1/1

== system LMS_cs/BMW_X5_SUV_8/Dynamics_Simple_3D/Chassis/Bicycle_model_[XYZ]/Z, Pitch_Motion & Roll_Motion/Configurable Subsystem5 ==
  In1 : Inport
  Derivative : Derivative
  Out1 : Outport
  wires:
  In1/1 -> Derivative/1
  Derivative/1 -> Out1/1

== system LMS_cs/BMW_X5_SUV_8/Dynamics_Simple_3D/Chassis/Bicycle_model_[XYZ]/Z, Pitch_Motion & Roll_Motion/Configurable Subsystem6 ==
  In1 : Inport
  Derivative : Derivative
  Out1 : Outport
  wires:
  In1/1 -> Derivative/1
  Derivative/1 -> Out1/1

== system LMS_cs/BMW_X5_SUV_8/Dynamics_Simple_3D/Chassis/Bicycle_model_[XYZ]/Z, Pitch_Motion & Roll_Motion/Configurable Subsystem7 ==
  In1 : Inport
  Derivative : Derivative
  Out1 : Outport
  wires:
  In1/1 -> Derivative/1
  Derivative/1 -> Out1/1

== system LMS_cs/BMW_X5_SUV_8/Dynamics_Simple_3D/Chassis/Bicycle_model_[XYZ]/Z, Pitch_Motion & Roll_Motion/Configurable Subsystem8 ==
  In1 : Inport
  Derivative : Derivative
  Out1 : Outport
  wires:
  In1/1 -> Derivative/1
  Derivative/1 -> Out1/1

== system LMS_cs/BMW_X5_SUV_8/Dynamics_Simple_3D/Chassis/Bicycle_model_[XYZ]/Z, Pitch_Motion & Roll_Motion/Configurable Subsystem9 ==
  In1 : Inport
  Derivative : Derivative
  Out1 : Outport
  wires:
  In1/1 -> Derivative/1
  Derivative/1 -> Out1/1

== system LMS_cs/BMW_X5_SUV_8/Dynamics_Simple_3D/Chassis/Bicycle_model_[XYZ]/Z_Motion unsprung mass/Configurable Subsystem ==
  In1 : Inport
  Derivative : Derivative
  Out1 : Outport
  wires:
  In1/1 -> Derivative/1
  Derivative/1 -> Out1/1

== system LMS_cs/BMW_X5_SUV_8/Dynamics_Simple_3D/Chassis/Bicycle_model_[XYZ]/Z_Motion unsprung mass/Configurable Subsystem1 ==
  In1 : Inport
  Integrator : Integrator
  Out1 : Outport
  wires:
  In1/1 -> Integrator/1
  Integrator/1 -> Out1/1

== system LMS_cs/BMW_X5_SUV_8/Dynamics_Simple_3D/Chassis/Bicycle_model_[XYZ]/Z_Motion unsprung mass/Configurable Subsystem10 ==
  In1 : Inport
  Derivative : Derivative
  Out1 : Outport
  wires:
  In1/1 -> Derivative/1
  Derivative/1 -> Out1/1

== system LMS_cs/BMW_X5_SUV_8/Dynamics_Simple_3D/Chassis/Bicycle_model_[XYZ]/Z_Motion unsprung mass/Configurable Subsystem11 ==
  In1 : Inport
  Derivative : Derivative
  Out1 : Outport
  wires:
  In1/1 -> Derivative/1
  Derivative/1 -> Out1/1

== system LMS_cs/BMW_X5_SUV_8/Dynamics_Simple_3D/Chassis/Bicycle_model_[XYZ]/Z_Motion unsprung mass/Configurable Subsystem2 ==
  In1 : Inport
  Integrator : Integrator
  Out1 : Outport
  wires:
  In1/1 -> Integrator/1
  Integrator/1 -> Out1/1

== system LMS_cs/BMW_X5_SUV_8/Dynamics_Simple_3D/Chassis/Bicycle_model_[XYZ]/Z_Motion unsprung mass/Configurable Subsystem3 ==
  In1 : Inport
  Integrator : Integrator
  Out1 : Outport
  wires:
  In1/1 -> Integrator/1
  Integrator/1 -> Out1/1

== system LMS_cs/BMW_X5_SUV_8/Dynamics_Simple_3D/Chassis/Bicycle_model_[XYZ]/Z_Motion unsprung mass/Configurable Subsystem4 ==
  In1 : Inport
  Integrator : Integrator
  Out1 : Outport
  wires:
  In1/1 -> Integrator/1
  Integrator/1 -> Out1/1

== system LMS_cs/BMW_X5_SUV_8/Dynamics_Simple_3D/Chassis/Bicycle_model_[XYZ]/Z_Motion unsprung mass/Configurable Subsystem5 ==
  In1 : Inport
  Integrator : Integrator
  Out1 : Outport
  wires:
  In1/1 -> Integrator/1
  Integrator/1 -> Out1/1

== system LMS_cs/BMW_X5_SUV_8/Dynamics_Simple_3D/Chassis/Bicycle_model_[XYZ]/Z_Motion unsprung mass/Configurable Subsystem6 ==
  In1 : Inport
  Integrator : Integrator
  Out1 : Outport
  wires:
  In1/1 -> Integrator/1
  Integrator/1 -> Out1/1

== system LMS_cs/BMW_X5_SUV_8/Dynamics_Simple_3D/Chassis/Bicycle_model_[XYZ]/Z_Motion unsprung mass/Configurable Subsystem7 ==
  In1 : Inport
  Integrator : Integrator
  Out1 : Outport
  wires:
  In1/1 -> Integrator/1
  Integrator/1 -> Out1/1

== system LMS_cs/BMW_X5_SUV_8/Dynamics_Simple_3D/Chassis/Bicycle_model_[XYZ]/Z_Motion unsprung mass/Configurable Subsystem8 ==
  In1 : Inport
  Integrator : Integrator
  Out1 : Outport
  wires:
  In1/1 -> Integrator/1
  Integrator/1 -> Out1/1

== system LMS_cs/BMW_X5_SUV_8/Dynamics_Simple_3D/Chassis/Bicycle_model_[XYZ]/Z_Motion unsprung mass/Configurable Subsystem9 ==
  In1 : Inport
  Derivative : Derivative
  Out1 : Outport
  wires:
  In1/1 -> Derivative/1
  Derivative/1 -> Out1/1

== system LMS_cs/BMW_X5_SUV_8/Dynamics_Simple_3D/Chassis/FrontTyre/AlphaFront/Enabled Subsystem ==
  In : Inport
  Enable : EnablePort  PropagateVarSize=During execution
  AlphaFront : Fcn  Expr=-atan( (u(2)+u(3)*p.a)/u(1) )
  Alpha : Outport  OutputWhenDisabled=reset  InitialOutput=[0]
  wires:
  AlphaFront/1 -> Alpha/1
  In/1 -> AlphaFront/1

== system LMS_cs/BMW_X5_SUV_8/Dynamics_Simple_3D/Chassis/RearTyre/AlphaRear/Enabled Subsystem ==
  In : Inport
  Enable : EnablePort  PropagateVarSize=During execution
  AlphaRear : Fcn  Expr=-atan( (u(2)-u(3)*p.b)/u(1) )
  Alpha : Outport  OutputWhenDisabled=reset  InitialOutput=[0]
  wires:
  AlphaRear/1 -> Alpha/1
  In/1 -> AlphaRear/1

== system LMS_cs/BMW_X5_SUV_8/PreScan_Contact_Sensor/Vehicle Local to World/state2FullState/limit roll/Substitute 90 & 270 deg (and its plurals) ==
  Angle [rad] : Inport
  270 deg detection : simulink/Model Verification/Check  Static Gap  Description=u <= 269.5 || 270.5 <= u  max=270.5  max_included=on  min=269.5  min_included=on  enabled=on  stopWhenAssertionFail=off  export=on  icon=graphic
  90 deg detection : simulink/Model Verification/Check  Static Gap  Description=u <= 89.5 || 90.5 <= u  max=90.5  max_included=on  min=89.5  min_included=on  enabled=on  stopWhenAssertionFail=off  export=on  icon=graphic
  Angle 0-360 deg limiter : Subsystem
  Degrees to Radians : simulink_extras/Transformations/Degrees to Radians
  Radians to Degrees : simulink_extras/Transformations/Radians to Degrees
  Substitution Value : Constant  Value=269.5
  Substitution Value : Constant  Value=89.5
  Switch : Switch  Threshold=0.5  SaturateOnIntegerOverflow=off  InputSameDT=off
  Switch1 : Switch  Threshold=0.5  SaturateOnIntegerOverflow=off  InputSameDT=off
  Subst Angle [rad] : Outport
  wires:
  Angle [rad]/1 -> Radians to Degrees/1
  Degrees to Radians/1 -> Subst Angle [rad]/1
  Radians to Degrees/1 -> Angle 0-360 deg limiter/1(Angle [deg])
  Switch1/1 -> Degrees to Radians/1
  Substitution Value/1 -> Switch1/3
  270 deg detection/1 -> Switch1/2
  Switch/1 -> Switch1/1, 270 deg detection/1
  Substitution Value/1 -> Switch/3
  90 deg detection/1 -> Switch/2
  Angle 0-360 deg limiter/1(LimAngle [deg]) -> 90 deg detection/1, Switch/1

== system LMS_cs/BMW_X5_SUV_9/Dynamics_Simple_3D/Chassis/Bicycle_model_[XYZ]/RoadContact/Penetration depth ==
  TyreInfo_in : Inport
  Bus Selector1 : BusSelector  OutputSignals=TireFL.cp0.penetrationdepth,TireFL.cp0.normal.z,TireFL.cp1.penetrationdepth,TireFL.cp1.normal.z,TireFL.cp2.penetrationdepth,TireFL.cp2.normal.z,TireFL.cp3.penetrationdepth,TireFL.cp3.normal.z,TireFR.cp0.penetrationdepth,TireFR.cp0.normal.z,TireFR.cp1.penetrationdepth,TireFR.cp1.normal.z,TireFR.cp2.penetrationdepth,TireFR.cp2.normal.z,TireFR.cp3.penetrationdepth,TireFR.cp3.normal.z,TireRL.cp0.penetrationdepth,TireRL.cp0.normal.z,TireRL.cp1.penetrationdepth,TireRL.cp1.normal.z,TireRL.cp2.penetrationdepth,TireRL.cp2.normal.z,TireRL.cp3.penetrationdepth,TireRL.cp3.normal.z,TireRR.cp0.penetrationdepth,TireRR.cp0.normal.z,TireRR.cp1.penetrationdepth,TireRR.cp1.normal.z,TireRR.cp2.penetrationdepth,TireRR.cp2.normal.z,TireRR.cp3.penetrationdepth,TireRR.cp3.normal.z
  Fcn{,1..15} (16 alike) : Fcn  Expr=u(1)*u(2)
  MinMax{1..4} (4 alike) : MinMax
  Mux{1..4} (4 alike) : Mux
  Mux{5..20} (16 alike) : Mux  Inputs=2
  Saturation{1..4} (4 alike) : Saturate  UpperLimit=0  LowerLimit=-inf
  depth_FL [m] : Outport
  depth_FR [m] : Outport  Port=2
  depth_RL [m] : Outport  Port=3
  depth_RR [m] : Outport  Port=4
  wires:
  Fcn15/1 -> Mux4/4
  Fcn14/1 -> Mux4/3
  Fcn13/1 -> Mux4/2
  Fcn12/1 -> Mux4/1
  Fcn11/1 -> Mux2/4
  Fcn10/1 -> Mux2/3
  Fcn9/1 -> Mux2/2
  Fcn8/1 -> Mux2/1
  Mux15/1 -> Fcn15/1
  Mux14/1 -> Fcn14/1
  Mux13/1 -> Fcn13/1
  Mux20/1 -> Fcn12/1
  Mux19/1 -> Fcn11/1
  Mux18/1 -> Fcn10/1
  Mux17/1 -> Fcn9/1
  Mux16/1 -> Fcn8/1
  Fcn7/1 -> Mux1/4
  Fcn6/1 -> Mux1/3
  Fcn5/1 -> Mux1/2
  Fcn4/1 -> Mux1/1
  Fcn3/1 -> Mux3/4
  Fcn2/1 -> Mux3/3
  Fcn1/1 -> Mux3/2
  Fcn/1 -> Mux3/1
  Mux12/1 -> Fcn7/1
  Mux11/1 -> Fcn6/1
  Mux10/1 -> Fcn5/1
  Mux9/1 -> Fcn4/1
  Mux8/1 -> Fcn3/1
  Mux7/1 -> Fcn2/1
  Mux6/1 -> Fcn1/1
  Mux5/1 -> Fcn/1
  MinMax1/1 -> Saturation2/1
  Mux1/1 -> MinMax1/1
  MinMax2/1 -> Saturation3/1
  Mux2/1 -> MinMax2/1
  MinMax4/1 -> Saturation1/1
  Bus Selector1/32 -> Mux15/2  "<z>"
  Bus Selector1/31 -> Mux15/1  "<penetrationdepth>"
  Bus Selector1/30 -> Mux14/2  "<z>"
  Bus Selector1/29 -> Mux14/1  "<penetrationdepth>"
  Bus Selector1/28 -> Mux13/2  "<z>"
  Bus Selector1/27 -> Mux13/1  "<penetrationdepth>"
  Bus Selector1/26 -> Mux20/2  "<z>"
  Bus Selector1/25 -> Mux20/1  "<penetrationdepth>"
  Bus Selector1/24 -> Mux19/2  "<z>"
  Bus Selector1/23 -> Mux19/1  "<penetrationdepth>"
  Bus Selector1/22 -> Mux18/2  "<z>"
  Bus Selector1/21 -> Mux18/1  "<penetrationdepth>"
  Bus Selector1/20 -> Mux17/2  "<z>"
  Bus Selector1/19 -> Mux17/1  "<penetrationdepth>"
  Bus Selector1/18 -> Mux16/2  "<z>"
  Bus Selector1/17 -> Mux16/1  "<penetrationdepth>"
  Bus Selector1/16 -> Mux12/2  "<z>"
  Bus Selector1/15 -> Mux12/1  "<penetrationdepth>"
  Bus Selector1/14 -> Mux11/2  "<z>"
  Bus Selector1/13 -> Mux11/1  "<penetrationdepth>"
  Bus Selector1/12 -> Mux10/2  "<z>"
  Bus Selector1/11 -> Mux10/1  "<penetrationdepth>"
  Bus Selector1/10 -> Mux9/2  "<z>"
  Bus Selector1/9 -> Mux9/1  "<penetrationdepth>"
  Bus Selector1/8 -> Mux8/2  "<z>"
  Bus Selector1/7 -> Mux8/1  "<penetrationdepth>"
  Bus Selector1/6 -> Mux7/2  "<z>"
  Bus Selector1/5 -> Mux7/1  "<penetrationdepth>"
  Bus Selector1/4 -> Mux6/2  "<z>"
  Bus Selector1/3 -> Mux6/1  "<penetrationdepth>"
  Bus Selector1/2 -> Mux5/2  "<z>"
  Bus Selector1/1 -> Mux5/1  "<penetrationdepth>"
  Mux4/1 -> MinMax3/1
  MinMax3/1 -> Saturation4/1
  Mux3/1 -> MinMax4/1
  Saturation1/1 -> depth_FL [m]/1
  Saturation2/1 -> depth_FR [m]/1
  TyreInfo_in/1 -> Bus Selector1/1
  Saturation3/1 -> depth_RL [m]/1
  Saturation4/1 -> depth_RR [m]/1

== system LMS_cs/BMW_X5_SUV_9/Dynamics_Simple_3D/Chassis/Bicycle_model_[XYZ]/RoadContact/RoadGeometry ==
  TyreInfo_in : Inport
  Calc_banking : Subsystem
  Calc_slope : Subsystem
  Calc_z : Subsystem
  DocBlock : simulink/Model-Wide Utilities/DocBlock  DocumentType=Text
      content=|
      | This block determines, based on the z-coordinates of the road in
      | correspondence of the contact points,
      | - the z-coordinate of the road in correspondence of the middle point of the
      |   vehicle (z);
      | - the slope angle of the road (alpha, positive when downhill);
      | - the banking angle of the road (beta, positive when counter-clockwise when
      |   looking from the front of the vehicle).
      |
      | For every wheel there are 4 contact points (cp0, cp1, cp2, cp3) defined in
      | TyreInfo_in. Not all 4 contact points reports always a value, depending on
      | different conditions there might be contact points that do not report a
      | value. These points report in this case to 0. If the tyre is lifted from
      | the road, all contact points report 0. Because of this reason, the
      | value of the contact point that reports the largest negative value of the
      | penetration depth is used. If all values of the penetration depth are 0,
      | then a maximum gradient is applied to avoid jumps to 0 in the z signal.
      | The maximum gradient is fixed to -6 [m/s^2], this value is large enough for
      | a vehicle driving at 30 [m/s] downhill on a gradient of 20 [%]. Further, a
      | first order low pass linear filter with a bandwidth of 1 [Hz] is applied.
      | This filter removes high frequencies components in the signal, when one
      | wheel is lifted (e.g. drive in a corner with a large lateral acceleration).
      | The bandwidth of 1 [Hz] is large enough to include the main frequencies
      | that occurr in the vehicle roll, pitch and vertical movements.
      |
      | z, slope and banking are determined as follows:
      |
      | z        = (+ zFL + zFR + zRL + zRR) / 4            (Calc_z)
      | slope    = (- zFL - zFR + zRL + zRR) / (2*p.l)      (Calc_slope)
      | banking  = (+ zFL - zFR + zRL - zRR) / (2*p.width)  (Calc_banking)
  Mux4 : Mux
  zFL_lowerpenetrationdetph : Subsystem
  zFL_tyreinfo : Subsystem
  zFR_lowerpenetrationdetph : Subsystem
  zFR_tyreinfo : Subsystem
  zRL_lowerpenetrationdetph : Subsystem
  zRL_tyreinfo : Subsystem
  zRR_lowerpenetrationdetph : Subsystem
  zRR_tyreinfo : Subsystem
  z : Outport
  slope : Outport  Port=2
  banking : Outport  Port=3
  wires:
  TyreInfo_in/1 -> zFL_tyreinfo/1(In1), zFR_tyreinfo/1(In1), zRL_tyreinfo/1(In1), zRR_tyreinfo/1(In1)
  Calc_z/1(z) -> z/1
  Mux4/1 -> Calc_z/1(zi), Calc_slope/1(zi), Calc_banking/1(zi)
  Calc_slope/1(slope) -> slope/1
  Calc_banking/1(banking) -> banking/1
  zFL_lowerpenetrationdetph/1(z) -> Mux4/1
  zFR_lowerpenetrationdetph/1(z) -> Mux4/2
  zRL_lowerpenetrationdetph/1(z) -> Mux4/3
  zRR_lowerpenetrationdetph/1(z) -> Mux4/4
  zFL_tyreinfo/1(penetrationdepth) -> zFL_lowerpenetrationdetph/1(penetrationdepth)
  zFL_tyreinfo/2(position_z) -> zFL_lowerpenetrationdetph/2(position_z)
  zFL_tyreinfo/3(normal_z) -> zFL_lowerpenetrationdetph/3(normal_z)
  zFR_tyreinfo/1(penetrationdepth) -> zFR_lowerpenetrationdetph/1(penetrationdepth)
  zFR_tyreinfo/2(position_z) -> zFR_lowerpenetrationdetph/2(position_z)
  zFR_tyreinfo/3(normal_z) -> zFR_lowerpenetrationdetph/3(normal_z)
  zRL_tyreinfo/1(penetrationdepth) -> zRL_lowerpenetrationdetph/1(penetrationdepth)
  zRL_tyreinfo/2(position_z) -> zRL_lowerpenetrationdetph/2(position_z)
  zRL_tyreinfo/3(normal_z) -> zRL_lowerpenetrationdetph/3(normal_z)
  zRR_tyreinfo/1(penetrationdepth) -> zRR_lowerpenetrationdetph/1(penetrationdepth)
  zRR_tyreinfo/2(position_z) -> zRR_lowerpenetrationdetph/2(position_z)
  zRR_tyreinfo/3(normal_z) -> zRR_lowerpenetrationdetph/3(normal_z)

== system LMS_cs/BMW_X5_SUV_9/Dynamics_Simple_3D/Chassis/Bicycle_model_[XYZ]/X_Motion/Air&RoadResistance ==
  vx_[ms-1] : Inport
  slope_[rad] : Inport  Port=2
  Gain : Gain  Gain=1/p.Rw
  Mux4 : Mux  Inputs=2
  Road & Aerodyn Resistances : Fcn  Expr=p.Rroad*cos(u(2)) + p.Rair*u(1)^2
  Saturation1 : Saturate  UpperLimit=5/15  LowerLimit=-5/15
  Sign : Signum
  "[ms-1] 2 [rads-1]" : Gain  Gain=1/p.Rw  SaturateOnIntegerOverflow=on  OutDataTypeStr=Inherit: Same as input  ParamDataTypeStr=Inherit: Same as input
  signed load1 : Product  InputSameDT=on  SaturateOnIntegerOverflow=on  OutDataTypeStr=Inherit: Same as first input
  Resistance_Force : Outport
  wires:
  Gain/1 -> signed load1/1  "ResistanceForce_[N]"
  slope_[rad]/1 -> Mux4/2
  Mux4/1 -> Road & Aerodyn Resistances/1
  Road & Aerodyn Resistances/1 -> Gain/1  "ResistanceTorque_[Nm]"
  Sign/1 -> signed load1/2  "sign"
  "[ms-1] 2 [rads-1]"/1 -> Saturation1/1
  Saturation1/1 -> Sign/1
  vx_[ms-1]/1 -> Mux4/1, "[ms-1] 2 [rads-1]"/1
  signed load1/1 -> Resistance_Force/1  "F_[N]"

== system LMS_cs/BMW_X5_SUV_9/Dynamics_Simple_3D/Chassis/Bicycle_model_[XYZ]/X_Motion/BrakeSystem ==
  vx_[ms-1] : Inport
  BrakePressure_[bar] : Inport  Port=2
  Gain : Gain  Gain=1/p.Rw
  Saturation : Saturate  UpperLimit=p.PBrakeMax  LowerLimit=0
  Saturation1 : Saturate  UpperLimit=5/15  LowerLimit=-5/15
  Sign : Signum
  "[ms-1] 2 [rads-1]" : Gain  Gain=1/p.Rw  SaturateOnIntegerOverflow=on  OutDataTypeStr=Inherit: Same as input  ParamDataTypeStr=Inherit: Same as input
  braking Q factor : Gain  Gain=p.Qfac  SaturateOnIntegerOverflow=on  OutDataTypeStr=Inherit: Same as input  ParamDataTypeStr=Inherit: Same as input
  signed load1 : Product  InputSameDT=on  SaturateOnIntegerOverflow=on  OutDataTypeStr=Inherit: Same as first input
  BrakeForce : Outport
  BrakeTorqueAbs : Outport  Port=2
  wires:
  Gain/1 -> signed load1/1
  signed load1/1 -> BrakeForce/1
  Sign/1 -> signed load1/2  "sign"
  "[ms-1] 2 [rads-1]"/1 -> Saturation1/1
  Saturation1/1 -> Sign/1
  vx_[ms-1]/1 -> "[ms-1] 2 [rads-1]"/1
  Saturation/1 -> braking Q factor/1
  BrakePressure_[bar]/1 -> Saturation/1
  braking Q factor/1 -> Gain/1, BrakeTorqueAbs/1

== system LMS_cs/BMW_X5_SUV_9/Dynamics_Simple_3D/Chassis/Bicycle_model_[XYZ]/X_Motion/Configurable Subsystem ==
  In1 : Inport
  In2 : Inport  Port=2
  In3 : Inport  Port=3
  Integrator : Integrator  ExternalReset=level  InitialConditionSource=external
  Out1 : Outport
  wires:
  In1/1 -> Integrator/1
  In2/1 -> Integrator/2
  In3/1 -> Integrator/3
  Integrator/1 -> Out1/1

== system LMS_cs/BMW_X5_SUV_9/Dynamics_Simple_3D/Chassis/Bicycle_model_[XYZ]/X_Motion/Configurable Subsystem1 ==
  In1 : Inport
  Torsional damping : TransferFcn  Denominator=[0.1 1]
  Out1 : Outport
  wires:
  In1/1 -> Torsional damping/1
  Torsional damping/1 -> Out1/1
